simulink model "TestLib"  (R2019a)
settings: Solver=FixedStepDiscrete  StartTime=0.0  StopTime=inf  FixedStep=0.1  RelTol=1e-3
libraries: Library x7
settings Model: Creator=Konstantin  LastModifiedBy=Konstantin
settings DebuggingCC: BusObjectLabelMismatch=error
settings ConfigComp: PLC_RTWSimulinkBlockComments=off  PLC_TargetIDE=tiaportal  PLC_GenerateReusableCode=on  PLC_ReuseMLFcnVariable=on  PLC_FBUseSubsystemInstanceName=on  PLC_PLCEnableBlockDescription=off  PLC_GenerateReport=off  PLC_LaunchReport=off

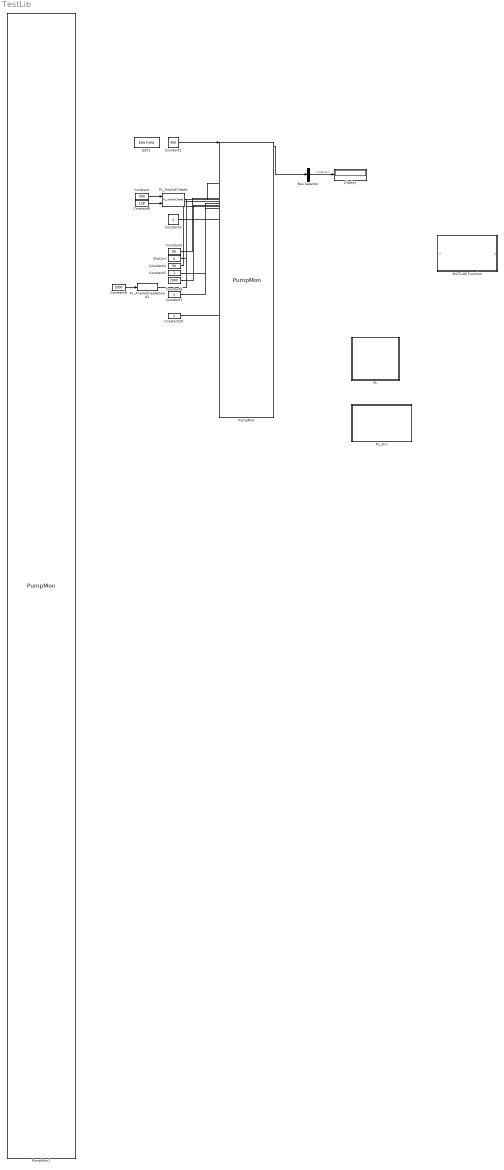
== system TestLib ==
  Bus Selector : BusSelector  OutputSignals=Value
  Constant : Constant  Value=390
  Constant1 : Constant  Value=400
  Constant{3,5,7,10} (4 alike) : Constant
  Constant2 : Constant  Value=80
  Constant4 : Constant  Value=50
  Constant6 : Constant  Value=2900
  Constant8 : Constant  Value=1000
  Constant9 : Constant  Value=128  OutDataTypeStr=int16
  Display : Display
  Edit1 : EditField  LabelPosition=Hide  ShowInitialText=on  Alignment=Center
  MATLAB Function : MATLAB Function  TreatAsAtomicUnit=on
  PL : Subsystem  TreatAsAtomicUnit=on
  PL_AnaValCreate : Library/Channel/PL_AnaValCreate  SystemSampleTime=-1
  PL_AnaValCreateGood1 : Library/Channel/PL_AnaValCreateGood  SystemSampleTime=-1
  PL_Sim : Subsystem
  PumpMon : Library/Condition Monitoring/PumpMon  SystemSampleTime=-1
  PumpMon1 : Library/Condition Monitoring/PumpMon  SystemSampleTime=-1
  SlipCorr : Constant  Value=0  OutDataTypeStr=boolean
  wires:
  Bus Selector/1 -> Display/1  "<Value>"
  PumpMon/1 -> Bus Selector/1
  Constant/1 -> PL_AnaValCreate/1
  Constant1/1 -> PumpMon/1
  Constant3/1 -> ?
  SlipCorr/1 -> ?
  Constant2/1 -> ?
  Constant4/1 -> ?
  Constant5/1 -> ?
  Constant6/1 -> ?
  Constant7/1 -> ?
  PL_AnaValCreateGood1/1 -> ?
  Constant8/1 -> PL_AnaValCreateGood1/1
  PL_AnaValCreate/1 -> ?
  Constant9/1 -> PL_AnaValCreate/2
  Constant10/1 -> ?

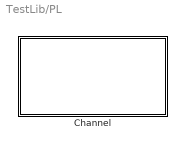
== system TestLib/PL ==
  Channel : Subsystem  TreatAsAtomicUnit=on
      settings: RTWFcnNameOpts=Use subsystem name  RTWFileNameOpts=Use subsystem name

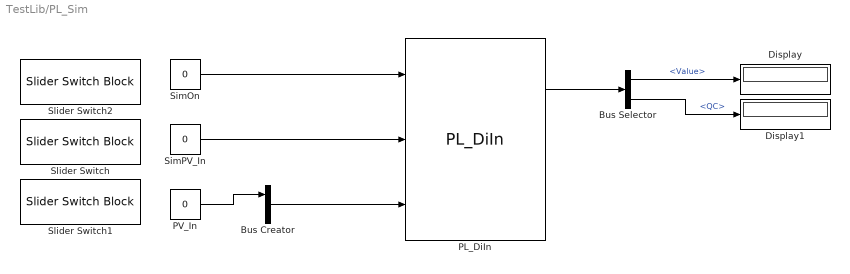
== system TestLib/PL_Sim ==
  Bus Creator : BusCreator  Inputs=2  OutDataTypeStr=Bus: DigValRaw
      settings: InheritFromInputs=off
  Bus Selector : BusSelector  OutputSignals=Value,QC
  Display : Display
  Display1 : Display
  PL_DiIn : Library/Channel/PL_DiIn  SystemSampleTime=-1
  PV_In : Constant  Value=0  OutDataTypeStr=boolean
  SimOn : Constant  Value=0  OutDataTypeStr=boolean
  SimPV_In : Constant  Value=0  OutDataTypeStr=boolean
  Slider Switch : SliderSwitchBlock
      settings: Values={{'Off', 'On'}, [0 1]}
  Slider Switch1 : SliderSwitchBlock
      settings: Values={{'Off', 'On'}, [0 1]}
  Slider Switch2 : SliderSwitchBlock
      settings: Values={{'Off', 'On'}, [0 1]}
  wires:
  SimPV_In/1 -> PL_DiIn/2
  Bus Creator/1 -> PL_DiIn/3
  PV_In/1 -> Bus Creator/1
  PL_DiIn/1 -> Bus Selector/1
  Bus Selector/1 -> Display/1  "<Value>"
  Bus Selector/2 -> Display1/1  "<QC>"
  SimOn/1 -> PL_DiIn/1

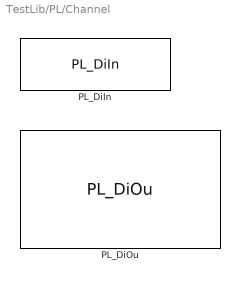
== system TestLib/PL/Channel ==
  PL_DiIn : Library/Channel/PL_DiIn  SystemSampleTime=-1
  PL_DiOu : Library/Channel/PL_DiOu  SystemSampleTime=-1

== matlab function TestLib/MATLAB Function ==
  data: u input; y output
function y = fcn(u)
%#codegen

y = subfunc(u);

function suby = subfunc(x)
suby = x * x;
